simulink model "Factorial"  (R2021a)
settings: Solver=FixedStepAuto  StartTime=0.0  StopTime=10.0  RelTol=1e-3
settings Model: Creator=user  LastModifiedBy=user
settings OptimizationCC: DefaultParameterBehavior=Inlined  EnhancedBackFolding=on  PassReuseOutputArgsAs=Individual arguments  ZeroExternalMemoryAtStartup=off  ZeroInternalMemoryAtStartup=off  OptimizeBlockOrder=speed  DifferentSizesBufferReuse=on  OptimizationCustomize=off  EfficientTunableParamExpr=on
settings DebuggingCC: ParameterTunabilityLossMsg=error
settings SFSimCC: MATLABDynamicMemAlloc=off
settings RTWCC: SystemTargetFile=ert.tlc  GenCodeOnly=on  TemplateMakefile=ert_default_tmf  GenerateReport=on  IncludeHyperlinkInReport=on  LaunchReport=on  GenerateTraceInfo=on
settings CodeAppCC: ForceParamTrailComments=on  IgnoreCustomStorageClasses=off  OperatorAnnotations=on  SimulinkDataObjDesc=on  SFDataObjDesc=on  InsertBlockDesc=on
settings ERTTargetCC: TargetLangStandard=C99 (ISO)  GenerateSampleERTMain=on  InlinedParameterPlacement=NonHierarchical  ERTCustomFileTemplate=example_file_process.tlc

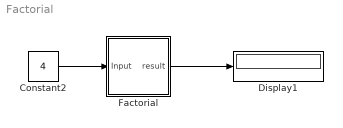
== system Factorial ==
  Constant2 : Constant  Value=4  OutDataTypeStr=uint16
  Display1 : Display
  Factorial : Stateflow chart  TreatAsAtomicUnit=on
  wires:
  Constant2/1 -> Factorial/1(Input)
  Factorial/1(result) -> Display1/1

== stateflow chart Factorial/Factorial ==
  (default) -> (junction 9)
  (junction 9) -> (junction 11)
  (junction 11) -> (junction 10) [order 1] : [index<=Input]
  (junction 12) -> (junction 11)
  (junction 10) -> (junction 12) : {result= index *result;
      |  index++ ; }
  (junction 11) -> (junction 13) [order 2]
  data: Input input uint16; result output uint16 =1; index local uint16 =1
